simulink library "libc_hmi"  (R2015b)
settings: Solver=ode45  StartTime=0.0  StopTime=10.0  RelTol=1e-3
undefined symbols (not defined in the file or in its folder): CONST, CTRL, DiscIntNeverNeededParam
libraries: simulink x10, libc_extended_basics x4, libc_filters_diff x2
settings Model: Creator=Falkenhahn  LastModifiedBy=fav
settings DataIOCC: SaveFormat=Array  SignalLoggingSaveFormat=ModelDataLogs
settings OptimizationCC: ExpressionDepthLimit=2147483647
settings DebuggingCC: UnderspecifiedInitializationDetection=Classic  MergeDetectMultiDrivingBlocksExec=none  SolverPrmCheckMsg=warning  FcnCallInpInsideContextMsg=UseLocalSettings  StateNameClashWarn=warning
settings HardwareCC: ProdBitPerPointer=32  ProdLargestAtomicFloat=None  ProdIntDivRoundTo=Undefined  ProdEndianess=Unspecified  ProdWordSize=32  ProdHWDeviceType=32-bit Generic
settings GRTTargetCC: GeneratePreprocessorConditionals=Disable all  CombineOutputUpdateFcns=off  GRTInterface=on
settings ConfigComp: CovModelRefEnable=Off

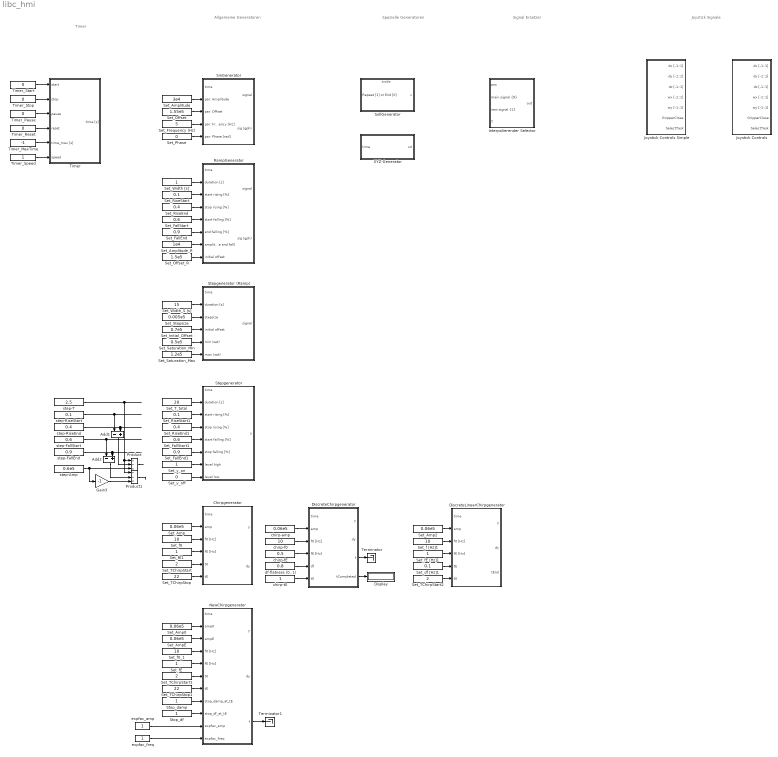
== system libc_hmi ==
  note: Timer
  note: Allgemeine
      | Generatoren
  note: Spezielle
      | Generatoren
  note: Signal
      | Ersetzer
  note: Joystick
      | Signale
  Add1 : Sum  Inputs=-+
  Add2 : Sum  Inputs=-+
  Chirpgenerator : Subsystem
      settings: AttributesFormatString=[f0,fE] >> 1/(tE-t0)
  DiscreteChirpgenerator : Subsystem
  DiscreteLinearChirpgenerator : Subsystem
  Display : Display
  Gain3 : Gain  Gain=-1
  Interpolierender Selector : Subsystem
  Joystick Controls : Subsystem  TreatAsAtomicUnit=on  SystemSampleTime=CONST.tA
      settings: AttributesFormatString=|
      | Neues Mapping mit Entprellung für BluetoothController
      | -- beachte entsprechende Einstellungen in ControlDesk --
  Joystick Controls Simple : Subsystem  TreatAsAtomicUnit=on  SystemSampleTime=CONST.tA
      settings: AttributesFormatString=|
      | Neues Mapping
      | -- beachte entsprechende --
      | -- Einstellungen in ControlDesk --
  NewChirpgenerator : Subsystem
  Product : Product  Inputs=//*
  Product1 : Product  Inputs=//*
  RampGenerator : Subsystem
  Set_Amp : Constant  Value=0.06e5
  Set_Amp0 : Constant  Value=0.06e5
  Set_Amp2 : Constant  Value=0.06e5
  Set_AmpE : Constant  Value=0.06e5
  Set_Amplitude : Constant  Value=3e4
  Set_Amplitude_R : Constant  Value=1e4
  Set_FallEnd : Constant  Value=0.9
  Set_FallEnd1 : Constant  Value=0.9
  Set_FallStart : Constant  Value=0.6
  Set_FallStart1 : Constant  Value=0.6
  Set_Frequency (Hz) : Constant  Value=5
  Set_Initial_Offset : Constant  Value=0.7e5
  Set_Offset : Constant  Value=1.55e5
  Set_Offset_R : Constant  Value=1.5e5
  Set_Phase : Constant  Value=0
  Set_RiseEnd : Constant  Value=0.4
  Set_RiseEnd1 : Constant  Value=0.4
  Set_RiseStart : Constant  Value=0.1
  Set_RiseStart1 : Constant  Value=0.1
  Set_Saturation_Max : Constant  Value=1.2e5
  Set_Saturation_Min : Constant  Value=0.5e5
  Set_Stepsize : Constant  Value=0.005e5
  Set_TChirpStart : Constant  Value=2
  Set_TChirpStart1 : Constant  Value=2
  Set_TChirpStart2 : Constant  Value=2
  Set_TChirpStop : Constant  Value=22
  Set_TChirpStop1 : Constant  Value=22
  Set_T_total : Constant  Value=20
  Set_Width [s] : Constant
  Set_Width_S [s] : Constant  Value=15
  Set_df [Hz]1 : Constant  Value=0.1
  Set_f [Hz]1 : Constant  Value=10
  Set_f0 : Constant  Value=10
  Set_f0_1 : Constant  Value=10
  "Set_fE " : Constant
  Set_fE [Hz]1 : Constant
  "Set_fE1 " : Constant
  Set_y_off : Constant  Value=0
  Set_y_on : Constant
  SinGenerator : Subsystem
  SollGenerator : Subsystem  mask(zeitgesteuerter Interpolator){len_ti=length(CTRL.LPresetTime), repext_a=1, repext_z=1}
      mask prompts: len_ti "Datenpunkte (insg)"; repext_a "Startpunkte (vorne)"; repext_z "Endpunkte (hinten)"
      mask help: Anzahl Abtastpunkte, die vorne und hinten von der Wiederholung ausgenommen sind.
      mask init:
      | last_in_loop = len_ti - repext_z;
      | first_in_loop = 1 + repext_a;
  Stepgenerator : Subsystem
  Stepgenerator (Ramp) : Subsystem  mask{pulsewidth=40}
      mask prompts: pulsewidth "Pulse width [%]"
      settings: AttributesFormatString=Puls: 0 bis %<pulsewidth> %
  Stop_damp : Constant
  Stop_df : Constant
  Terminator : Terminator
  Terminator1 : Terminator
  Timer : Subsystem
  Timer_MaxTime : Constant  Value=-1
  Timer_Pause : Constant  Value=0
  Timer_Reset : Constant  Value=0
  Timer_Speed : Constant
  Timer_Start : Constant  Value=0
  Timer_Stop : Constant  Value=0
  XYZ-Generator : Subsystem
  chirp-amp : Constant  Value=0.06e5
  chirp-f0 : Constant  Value=10
  chirp-fE : Constant  Value=0.5
  chirp-t0 : Constant
  df-flatness (0..1) : Constant  Value=0.8
  expfac_amp : Constant
      settings: AttributesFormatString=|
      | > 0.1
      | 0.5 = sqrt
      | 1 = linear
      | 2 = quadratic
  expfac_freq : Constant
      settings: AttributesFormatString=|
      | > 0.1
      | 0.5 = sqrt
      | 1 = linear
      | 2 = quadratic
  step-Amp : Constant  Value=0.6e5
  step-FallEnd : Constant  Value=0.9
  step-FallStart : Constant  Value=0.6
  step-RiseEnd : Constant  Value=0.4
  step-RiseStart : Constant  Value=0.1
  step-T : Constant  Value=2.5
  wires:
  Set_Frequency (Hz)/1 -> SinGenerator/4(par: Frequency [Hz])
  Set_Phase/1 -> SinGenerator/5(par: Phase [rad])
  Set_Offset/1 -> SinGenerator/3(par: Offset)
  Set_Amplitude/1 -> SinGenerator/2(par: Amplitude)
  Set_Width [s]/1 -> RampGenerator/2(duration [s])
  Set_FallStart/1 -> RampGenerator/5(start falling [%])
  Set_RiseEnd/1 -> RampGenerator/4(stop rising [%])
  Set_RiseStart/1 -> RampGenerator/3(start rising [%])
  Set_Amplitude_R/1 -> RampGenerator/7(amplitude (rise and fall))
  Set_FallEnd/1 -> RampGenerator/6(end falling [%])
  Set_Offset_R/1 -> RampGenerator/8(initial offset)
  Set_Saturation_Max/1 -> Stepgenerator (Ramp)/6(max (sat))
  Set_Width_S [s]/1 -> Stepgenerator (Ramp)/2(duration [s])
  Set_Initial_Offset/1 -> Stepgenerator (Ramp)/4(initial offset)
  Set_Stepsize/1 -> Stepgenerator (Ramp)/3(stepsize)
  Set_Saturation_Min/1 -> Stepgenerator (Ramp)/5(min (sat))
  Set_y_on/1 -> Stepgenerator/7(level high)
  Set_y_off/1 -> Stepgenerator/8(level low)
  Set_T_total/1 -> Stepgenerator/2(duration [s])
  Set_RiseStart1/1 -> Stepgenerator/3(start rising [%])
  Set_RiseEnd1/1 -> Stepgenerator/4(stop rising [%])
  Set_FallStart1/1 -> Stepgenerator/5(start falling [%])
  Set_FallEnd1/1 -> Stepgenerator/6(stop falling [%])
  step-RiseStart/1 -> Add1/1
  step-RiseEnd/1 -> Add1/2
  step-FallStart/1 -> Add2/1
  step-FallEnd/1 -> Add2/2
  step-T/1 -> Product/1, Product1/1
  Add1/1 -> Product/2
  Add2/1 -> Product1/2
  step-Amp/1 -> Gain3/1, Product/3
  Gain3/1 -> Product1/3
  Product/1 -> ?
  Product1/1 -> ?
  Set_Amp/1 -> Chirpgenerator/2(amp)
  Set_f0/1 -> Chirpgenerator/3(f0 [Hz])
  "Set_fE1 "/1 -> Chirpgenerator/4(fE [Hz])
  Set_TChirpStart/1 -> Chirpgenerator/5(t0)
  Set_TChirpStop/1 -> Chirpgenerator/6(tE)
  Set_Amp2/1 -> DiscreteLinearChirpgenerator/2(amp)
  Set_fE [Hz]1/1 -> DiscreteLinearChirpgenerator/4(fE [Hz])
  Set_df [Hz]1/1 -> DiscreteLinearChirpgenerator/5(tE)
  Set_f [Hz]1/1 -> DiscreteLinearChirpgenerator/3(f0 [Hz])
  Set_TChirpStart2/1 -> DiscreteLinearChirpgenerator/6(t0)
  chirp-amp/1 -> DiscreteChirpgenerator/2(amp)
  chirp-f0/1 -> DiscreteChirpgenerator/3(f0 [Hz])
  chirp-fE/1 -> DiscreteChirpgenerator/4(fE [Hz])
  df-flatness (0..1)/1 -> DiscreteChirpgenerator/5(df)
  chirp-t0/1 -> DiscreteChirpgenerator/6(t0)
  DiscreteChirpgenerator/3(f) -> Terminator/1
  DiscreteChirpgenerator/4(tCompleted) -> Display/1
  Timer_Start/1 -> Timer/1(start)
  Timer_Reset/1 -> Timer/4(reset)
  Timer_Stop/1 -> Timer/2(stop)
  Timer_MaxTime/1 -> Timer/5(time_max [s])
  Timer_Pause/1 -> Timer/3(pause)
  Timer_Speed/1 -> Timer/6(speed)
  Set_TChirpStart1/1 -> NewChirpgenerator/6(t0)
  "Set_fE "/1 -> NewChirpgenerator/5(fE [Hz])
  Set_TChirpStop1/1 -> NewChirpgenerator/7(tE)
  Set_f0_1/1 -> NewChirpgenerator/4(f0 [Hz])
  Stop_df/1 -> NewChirpgenerator/9(stop_df_at_tE)
  Stop_damp/1 -> NewChirpgenerator/8(stop_damp_at_tE)
  Set_AmpE/1 -> NewChirpgenerator/3(ampE)
  Set_Amp0/1 -> NewChirpgenerator/2(amp0)
  expfac_amp/1 -> NewChirpgenerator/10(expfac_amp)
  expfac_freq/1 -> NewChirpgenerator/11(expfac_freq)
  NewChirpgenerator/3(f) -> Terminator1/1

== system libc_hmi/Chirpgenerator ==
  time : Inport
  amp : Inport  Port=2
  f0 [Hz] : Inport  Port=3
  fE [Hz] : Inport  Port=4
  t0 : Inport  Port=5
  tE : Inport  Port=6
  Gain1 : Gain  Gain=2*pi
  Gain2 : Gain  Gain=2*pi
  steps : MATLAB Function  TreatAsAtomicUnit=on
  y : Outport
  dy : Outport  Port=2
  wires:
  steps/2(dtsin) -> dy/1
  time/1 -> steps/1(time)
  amp/1 -> steps/2(amp)
  f0 [Hz]/1 -> Gain2/1
  fE [Hz]/1 -> Gain1/1
  t0/1 -> steps/5(t0)
  tE/1 -> steps/6(tE)
  Gain1/1 -> steps/4(wE)
  Gain2/1 -> steps/3(w0)
  steps/1(rsin) -> y/1

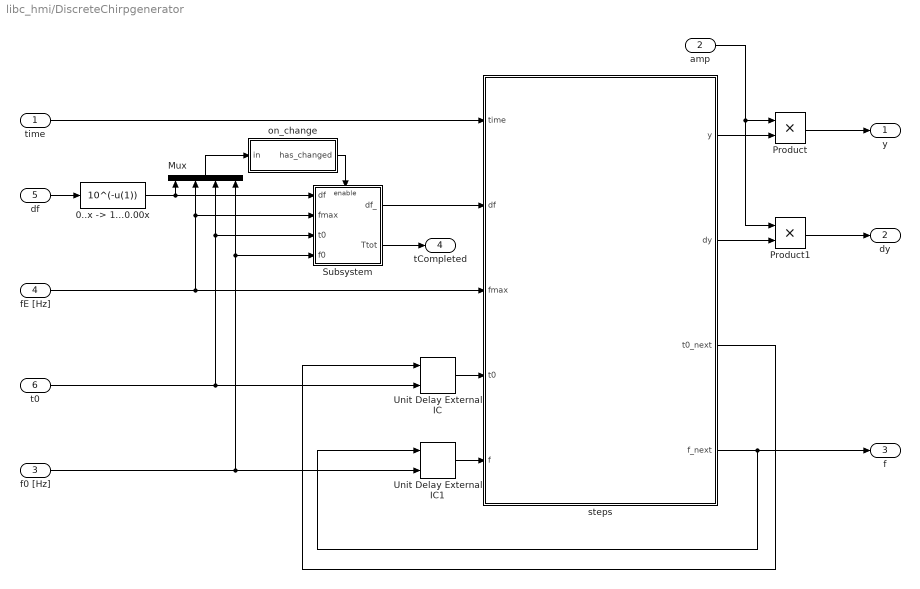
== system libc_hmi/DiscreteChirpgenerator ==
  time : Inport
  amp : Inport  Port=2
  f0 [Hz] : Inport  Port=3
  fE [Hz] : Inport  Port=4
  df : Inport  Port=5
  t0 : Inport  Port=6
  "0..x -> 1...0.00x" : Fcn  Expr=10^(-u(1))
  Mux : Mux
  Product : Product
  Product1 : Product
  Subsystem : Subsystem
  Unit Delay External IC : simulink/Additional Math & Discrete/Additional Discrete/Unit Delay External IC  tsamp=-1
  Unit Delay External IC1 : simulink/Additional Math & Discrete/Additional Discrete/Unit Delay External IC  tsamp=-1
  on_change : Subsystem
      settings: AttributesFormatString=|
      | from libl_filters_diff
      | variable frequency dependent filter
      | that has to be fixed
  steps : MATLAB Function  TreatAsAtomicUnit=on
  y : Outport
  dy : Outport  Port=2
  f : Outport  Port=3
  tCompleted : Outport  Port=4
  wires:
  "0..x -> 1...0.00x"/1 -> Mux/1, Subsystem/1(df)
  Mux/1 -> on_change/1(in)
  on_change/1(has_changed) -> Subsystem/Enable
  Subsystem/2(Ttot) -> tCompleted/1
  Subsystem/1(df_) -> steps/2(df)
  df/1 -> "0..x -> 1...0.00x"/1
  t0/1 -> Mux/3, Subsystem/3(t0), Unit Delay External IC/2
  steps/4(f_next) -> f/1, Unit Delay External IC1/1
  amp/1 -> Product1/1, Product/1
  Product1/1 -> dy/1
  steps/2(dy) -> Product1/2
  steps/1(y) -> Product/2
  fE [Hz]/1 -> Mux/2, Subsystem/2(fmax), steps/3(fmax)
  Unit Delay External IC1/1 -> steps/5(f)
  f0 [Hz]/1 -> Unit Delay External IC1/2, Mux/4, Subsystem/4(f0)
  Unit Delay External IC/1 -> steps/4(t0)
  steps/3(t0_next) -> Unit Delay External IC/1
  Product/1 -> y/1
  time/1 -> steps/1(time)

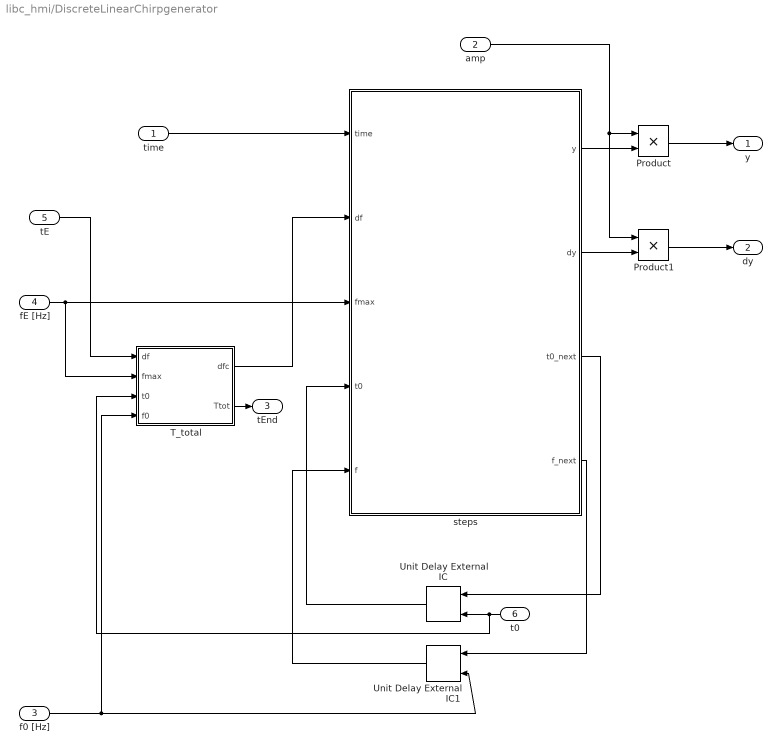
== system libc_hmi/DiscreteLinearChirpgenerator ==
  time : Inport
  amp : Inport  Port=2
  f0 [Hz] : Inport  Port=3
  fE [Hz] : Inport  Port=4
  tE : Inport  Port=5
  t0 : Inport  Port=6
  Product : Product
  Product1 : Product
  T_total : MATLAB Function  TreatAsAtomicUnit=on
  Unit Delay External IC : simulink/Additional Math & Discrete/Additional Discrete/Unit Delay External IC  tsamp=-1
  Unit Delay External IC1 : simulink/Additional Math & Discrete/Additional Discrete/Unit Delay External IC  tsamp=-1
  steps : MATLAB Function  TreatAsAtomicUnit=on
  y : Outport
  dy : Outport  Port=2
  tEnd : Outport  Port=3
  wires:
  time/1 -> steps/1(time)
  Product/1 -> y/1
  steps/3(t0_next) -> Unit Delay External IC/1
  Unit Delay External IC/1 -> steps/4(t0)
  t0/1 -> T_total/3(t0), Unit Delay External IC/2
  f0 [Hz]/1 -> T_total/4(f0), Unit Delay External IC1/2
  steps/4(f_next) -> Unit Delay External IC1/1
  Unit Delay External IC1/1 -> steps/5(f)
  tE/1 -> T_total/1(df)
  fE [Hz]/1 -> T_total/2(fmax), steps/3(fmax)
  steps/1(y) -> Product/2
  steps/2(dy) -> Product1/2
  Product1/1 -> dy/1
  amp/1 -> Product/1, Product1/1
  T_total/2(Ttot) -> tEnd/1
  T_total/1(dfc) -> steps/2(df)

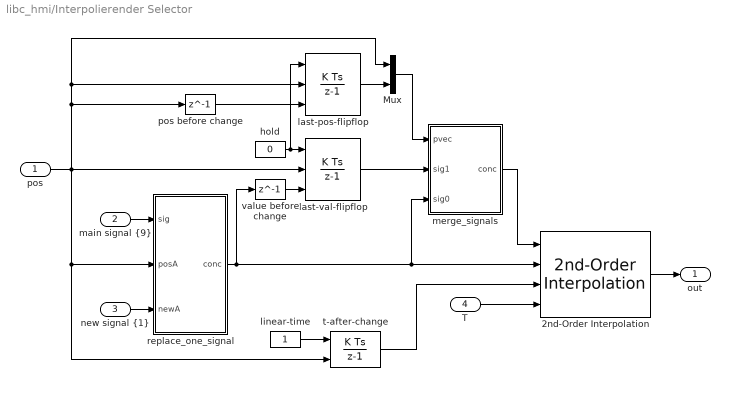
== system libc_hmi/Interpolierender Selector ==
  pos : Inport
  "main signal {9}" : Inport  Port=2
  "new signal {1}" : Inport  Port=3
  T : Inport  Port=4
  2nd-Order Interpolation : libc_filters_diff/2nd-Order Interpolation
  Mux : Mux  Inputs=2
  hold : Constant  Value=0
  last-pos-flipflop : DiscreteIntegrator  ExternalReset=either  InitialConditionSource=external  SampleTime=-1  ICPrevOutput=DiscIntNeverNeededParam  ICPrevScaledInput=DiscIntNeverNeededParam
  last-val-flipflop : DiscreteIntegrator  ExternalReset=either  InitialConditionSource=external  SampleTime=-1  ICPrevOutput=DiscIntNeverNeededParam  ICPrevScaledInput=DiscIntNeverNeededParam
  linear-time : Constant
  merge_signals : MATLAB Function  TreatAsAtomicUnit=on
  pos before change : Delay  DelayLength=1  InitialCondition=0
  replace_one_signal : MATLAB Function  TreatAsAtomicUnit=on
  t-after-change : DiscreteIntegrator  ExternalReset=either  InitialCondition=CONST.tA  SampleTime=-1  ICPrevOutput=DiscIntNeverNeededParam  ICPrevScaledInput=DiscIntNeverNeededParam
  value before change : Delay  DelayLength=1  InitialCondition=0.174
  out : Outport
  wires:
  "main signal {9}"/1 -> replace_one_signal/1(sig)
  "new signal {1}"/1 -> replace_one_signal/3(newA)
  replace_one_signal/1(conc) -> 2nd-Order Interpolation/2, merge_signals/3(sig0), value before change/1
  T/1 -> 2nd-Order Interpolation/4
  2nd-Order Interpolation/1 -> out/1
  pos/1 -> pos before change/1, last-pos-flipflop/2, Mux/1, t-after-change/2, replace_one_signal/2(posA), last-val-flipflop/2
  linear-time/1 -> t-after-change/1
  hold/1 -> last-pos-flipflop/1, last-val-flipflop/1
  value before change/1 -> last-val-flipflop/3
  last-val-flipflop/1 -> merge_signals/2(sig1)
  merge_signals/1(conc) -> 2nd-Order Interpolation/1
  t-after-change/1 -> 2nd-Order Interpolation/3
  Mux/1 -> merge_signals/1(pvec)
  last-pos-flipflop/1 -> Mux/2
  pos before change/1 -> last-pos-flipflop/3

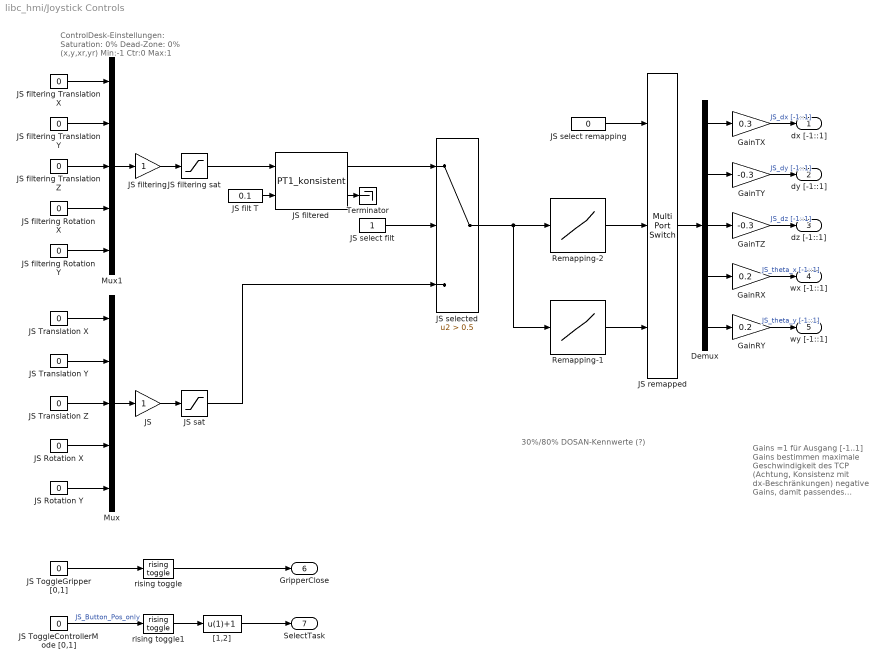
== system libc_hmi/Joystick Controls ==
  note: 30%/80% DOSAN-Kennwerte (?)
  note: Gains =1 für
      | Ausgang [-1..1]
      |
      | Gains bestimmen maximale
      | Geschwindigkeit des TCP
      | (Achtung, Konsistenz mit
      | dx-Beschränkungen)
      |
      | negative Gains,
      | damit passendes
      | Mapping für
      | stehendes
      | Welt-KoSy
  note: ControlDesk-Einstellungen:
      | Saturation: 0%
      | Dead-Zone: 0% (x,y,xr,yr)
      | Min:-1 Ctr:0 Max:1
  Demux : Demux  Outputs=5
  GainRX : Gain  Gain=0.2
  GainRY : Gain  Gain=0.2
  GainTX : Gain  Gain=0.3
  GainTY : Gain  Gain=-0.3
  GainTZ : Gain  Gain=-0.3
  JS : Gain
  JS Rotation X : Constant  Value=0  OutDataTypeStr=double
      settings: AttributesFormatString=[-1..1]
  JS Rotation Y : Constant  Value=0  OutDataTypeStr=double
      settings: AttributesFormatString=[-1..1]
  JS ToggleControllerMode [0,1] : Constant  Value=0  OutDataTypeStr=double
  JS ToggleGripper [0,1] : Constant  Value=0  OutDataTypeStr=double
  JS Translation X : Constant  Value=0  OutDataTypeStr=double
      settings: AttributesFormatString=[-1..1]
  JS Translation Y : Constant  Value=0  OutDataTypeStr=double
      settings: AttributesFormatString=[-1..1]
  JS Translation Z : Constant  Value=0  OutDataTypeStr=double
      settings: AttributesFormatString=[-1..1]
  JS filt T : Constant  Value=0.1
      settings: AttributesFormatString=|
      | 0.01: präzise, aber ruckartig
      | 0.1: weicher, dafür leicht verzögert
  JS filtered : libc_filters_diff/PT1_konsistent
  JS filtering : Gain
  JS filtering Rotation X : Constant  Value=0  OutDataTypeStr=double
      settings: AttributesFormatString=[-1..1]
  JS filtering Rotation Y : Constant  Value=0  OutDataTypeStr=double
      settings: AttributesFormatString=[-1..1]
  JS filtering Translation X : Constant  Value=0  OutDataTypeStr=double
      settings: AttributesFormatString=[-1..1]
  JS filtering Translation Y : Constant  Value=0  OutDataTypeStr=double
      settings: AttributesFormatString=[-1..1]
  JS filtering Translation Z : Constant  Value=0  OutDataTypeStr=double
      settings: AttributesFormatString=[-1..1]
  JS filtering sat : Saturate  UpperLimit=1  LowerLimit=-1
  JS remapped : MultiPortSwitch  DataPortOrder=Zero-based contiguous  Inputs=2
  JS sat : Saturate  UpperLimit=1  LowerLimit=-1
  JS select filt : Constant
      settings: AttributesFormatString=|
      | filtered input für
      | wireless controller
  JS select remapping : Constant  Value=0
  JS selected : Switch  Criteria=u2 > Threshold  Threshold=0.5
  Mux : Mux  Inputs=5
  Mux1 : Mux  Inputs=5
  Remapping-1 : Lookup_n-D  NumberOfTableDimensions=1  BreakpointsForDimension1="[-1, -0.9,  -0.301, -0.3, 0, 0.3, 0.301, 0.9, 1]"  Table=[-1, -1, -0.3, 0, 0, 0, 0.3, 1, 1]  InternalRulePriority=Speed  RndMeth=Simplest  InputSameDT=on
      settings: AttributesFormatString=|
      | Tote Zone mit
      | Losbrechsprung
      | und Plateau
  Remapping-2 : Lookup_n-D  NumberOfTableDimensions=1  BreakpointsForDimension1="[-1, -0.9,  -0.3, 0, 0.3, 0.9, 1]"  Table=[-1, -1, 0, 0, 0, 1, 1]  InternalRulePriority=Speed  RndMeth=Simplest  InputSameDT=on
      settings: AttributesFormatString=|
      | Tote Zone
      | mit Plateau
  Terminator : Terminator
  "[1,2]" : Fcn  Expr=u(1)+1
      settings: AttributesFormatString=toggle 1,2
  rising toggle : libc_extended_basics/rising toggle
  rising toggle1 : libc_extended_basics/rising toggle
  dx [-1::1] : Outport
  dy [-1::1] : Outport  Port=2
  dz [-1::1] : Outport  Port=3
  wx [-1::1] : Outport  Port=4
  wy [-1::1] : Outport  Port=5
  GripperClose : Outport  Port=6
  SelectTask : Outport  Port=7
      settings: AttributesFormatString=|
      | 0 off
      | 1 pos. only
      | 2 pos + orientation
  wires:
  JS selected/1 -> Remapping-2/1, Remapping-1/1
  JS select filt/1 -> JS selected/2
  JS sat/1 -> JS selected/3
  JS filtered/1 -> JS selected/1
  JS filtered/2 -> Terminator/1
  JS filt T/1 -> JS filtered/2
  JS filtering Translation Y/1 -> Mux1/2
  JS filtering Translation Z/1 -> Mux1/3
  JS filtering Rotation X/1 -> Mux1/4
  JS filtering Rotation Y/1 -> Mux1/5
  JS filtering sat/1 -> JS filtered/1
  JS filtering/1 -> JS filtering sat/1
  JS/1 -> JS sat/1
  Mux/1 -> JS/1
  Mux1/1 -> JS filtering/1
  JS filtering Translation X/1 -> Mux1/1
  JS Rotation Y/1 -> Mux/5
  JS Translation Y/1 -> Mux/2
  JS Translation Z/1 -> Mux/3
  JS Translation X/1 -> Mux/1
  JS Rotation X/1 -> Mux/4
  GainTX/1 -> dx [-1::1]/1  "JS_dx [-1::1]"
  GainTY/1 -> dy [-1::1]/1  "JS_dy [-1::1]"
  GainTZ/1 -> dz [-1::1]/1  "JS_dz [-1::1]"
  GainRX/1 -> wx [-1::1]/1  "JS_theta_x [-1::1]"
  GainRY/1 -> wy [-1::1]/1  "JS_theta_y [-1::1]"
  JS ToggleControllerMode [0,1]/1 -> rising toggle1/1  "JS_Button_Pos_only"
  JS ToggleGripper [0,1]/1 -> rising toggle/1
  "[1,2]"/1 -> SelectTask/1
  rising toggle/1 -> GripperClose/1
  rising toggle1/1 -> "[1,2]"/1
  Remapping-2/1 -> JS remapped/2
  Remapping-1/1 -> JS remapped/3
  JS select remapping/1 -> JS remapped/1
  JS remapped/1 -> Demux/1
  Demux/3 -> GainTZ/1
  Demux/2 -> GainTY/1
  Demux/4 -> GainRX/1
  Demux/1 -> GainTX/1
  Demux/5 -> GainRY/1

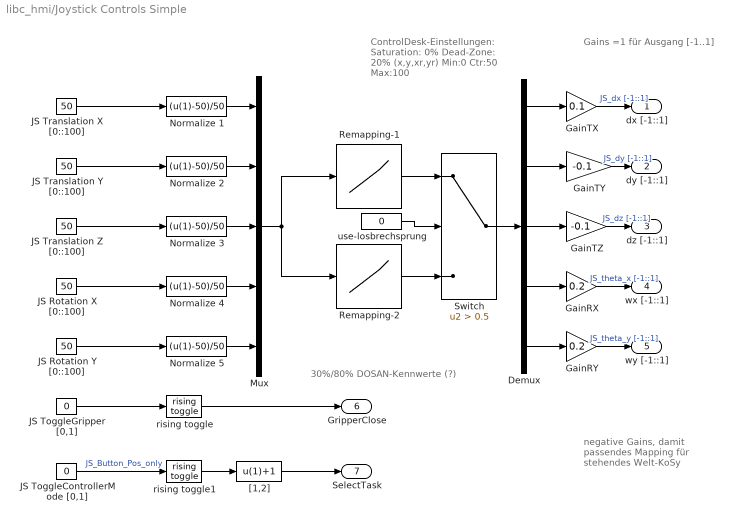
== system libc_hmi/Joystick Controls Simple ==
  note: 30%/80% DOSAN-Kennwerte (?)
  note: negative Gains,
      | damit passendes
      | Mapping für
      | stehendes
      | Welt-KoSy
  note: Gains =1 für
      | Ausgang [-1..1]
  note: ControlDesk-Einstellungen:
      | Saturation: 0%
      | Dead-Zone: 20% (x,y,xr,yr)
      | Min:0 Ctr:50 Max:100
  Demux : Demux  Outputs=5
  GainRX : Gain  Gain=0.2
  GainRY : Gain  Gain=0.2
  GainTX : Gain  Gain=0.1
  GainTY : Gain  Gain=-0.1
  GainTZ : Gain  Gain=-0.1
  JS Rotation X [0::100] : Constant  Value=50  OutDataTypeStr=double
  JS Rotation Y [0::100] : Constant  Value=50  OutDataTypeStr=double
  JS ToggleControllerMode [0,1] : Constant  Value=0  OutDataTypeStr=double
  JS ToggleGripper [0,1] : Constant  Value=0  OutDataTypeStr=double
  JS Translation X [0::100] : Constant  Value=50  OutDataTypeStr=double
  JS Translation Y [0::100] : Constant  Value=50  OutDataTypeStr=double
  JS Translation Z [0::100] : Constant  Value=50  OutDataTypeStr=double
  Mux : Mux  Inputs=5
  Normalize {1..5} (5 alike) : Fcn  Expr=(u(1)-50)/50
  Remapping-1 : Lookup_n-D  NumberOfTableDimensions=1  BreakpointsForDimension1="[-1, -0.9,  -0.301, -0.3, 0, 0.3, 0.301, 0.9, 1]"  Table=[-1, -1, -0.3, 0, 0, 0, 0.3, 1, 1]  InternalRulePriority=Speed  RndMeth=Simplest  InputSameDT=on
      settings: AttributesFormatString=|
      | Tote Zone mit
      | Losbrechsprung
      | und Plateau
  Remapping-2 : Lookup_n-D  NumberOfTableDimensions=1  BreakpointsForDimension1="[-1, -0.9,  -0.3, 0, 0.3, 0.9, 1]"  Table=[-1, -1, 0, 0, 0, 1, 1]  InternalRulePriority=Speed  RndMeth=Simplest  InputSameDT=on
      settings: AttributesFormatString=|
      | Tote Zone
      | mit Plateau
  Switch : Switch  Criteria=u2 > Threshold  Threshold=0.5
  "[1,2]" : Fcn  Expr=u(1)+1
      settings: AttributesFormatString=toggle 1,2
  rising toggle : libc_extended_basics/rising toggle
  rising toggle1 : libc_extended_basics/rising toggle
  use-losbrechsprung : Constant  Value=0
  dx [-1::1] : Outport
  dy [-1::1] : Outport  Port=2
  dz [-1::1] : Outport  Port=3
  wx [-1::1] : Outport  Port=4
  wy [-1::1] : Outport  Port=5
  GripperClose : Outport  Port=6
  SelectTask : Outport  Port=7
      settings: AttributesFormatString=|
      | 0 off
      | 1 pos. only
      | 2 pos + orientation
  wires:
  JS Translation X [0::100]/1 -> Normalize 1/1
  JS Translation Y [0::100]/1 -> Normalize 2/1
  JS Translation Z [0::100]/1 -> Normalize 3/1
  JS Rotation X [0::100]/1 -> Normalize 4/1
  JS Rotation Y [0::100]/1 -> Normalize 5/1
  GainTX/1 -> dx [-1::1]/1  "JS_dx [-1::1]"
  GainTY/1 -> dy [-1::1]/1  "JS_dy [-1::1]"
  GainTZ/1 -> dz [-1::1]/1  "JS_dz [-1::1]"
  GainRX/1 -> wx [-1::1]/1  "JS_theta_x [-1::1]"
  GainRY/1 -> wy [-1::1]/1  "JS_theta_y [-1::1]"
  JS ToggleControllerMode [0,1]/1 -> rising toggle1/1  "JS_Button_Pos_only"
  JS ToggleGripper [0,1]/1 -> rising toggle/1
  "[1,2]"/1 -> SelectTask/1
  rising toggle/1 -> GripperClose/1
  rising toggle1/1 -> "[1,2]"/1
  Normalize 3/1 -> Mux/3
  Normalize 2/1 -> Mux/2
  Normalize 4/1 -> Mux/4
  Normalize 1/1 -> Mux/1
  Normalize 5/1 -> Mux/5
  Mux/1 -> Remapping-1/1, Remapping-2/1
  Remapping-2/1 -> Switch/3
  Remapping-1/1 -> Switch/1
  use-losbrechsprung/1 -> Switch/2
  Switch/1 -> Demux/1
  Demux/3 -> GainTZ/1
  Demux/2 -> GainTY/1
  Demux/4 -> GainRX/1
  Demux/1 -> GainTX/1
  Demux/5 -> GainRY/1

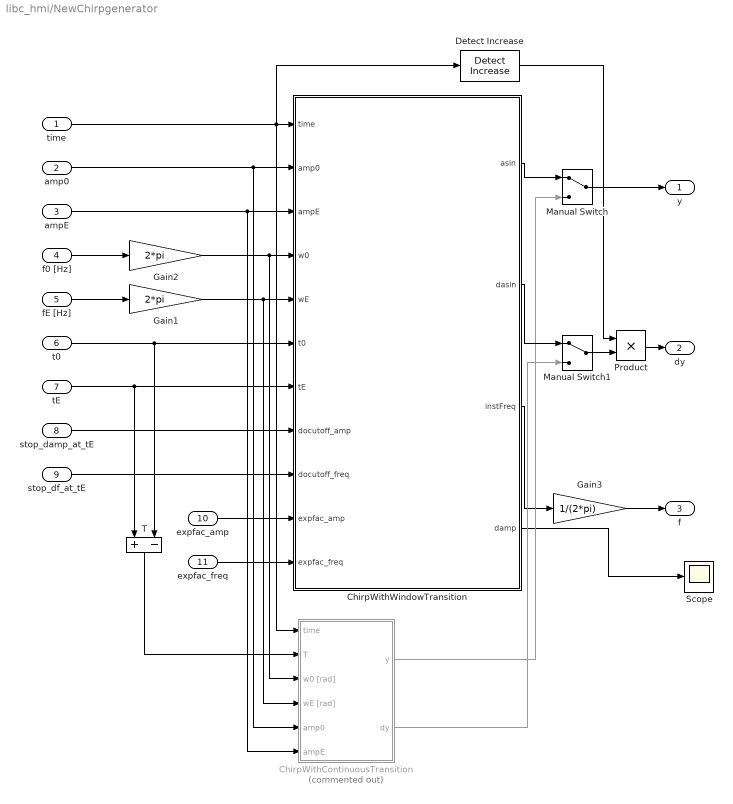
== system libc_hmi/NewChirpgenerator ==
  time : Inport
  amp0 : Inport  Port=2
  ampE : Inport  Port=3
  f0 [Hz] : Inport  Port=4
  fE [Hz] : Inport  Port=5
  t0 : Inport  Port=6
  tE : Inport  Port=7
  stop_damp_at_tE : Inport  Port=8
  stop_df_at_tE : Inport  Port=9
  expfac_amp : Inport  Port=10
  expfac_freq : Inport  Port=11
  ChirpWithContinuousTransition : Subsystem  Commented=on
  ChirpWithWindowTransition : MATLAB Function  TreatAsAtomicUnit=on
      settings: AttributesFormatString=allows: amp0=ampE & w0=wE
  Detect Increase : simulink/Logic and Bit Operations/Detect Increase  vinit=-1.0  InputProcessing=Inherited  OutDataTypeStr=boolean
  Gain1 : Gain  Gain=2*pi
  Gain2 : Gain  Gain=2*pi
  Gain3 : Gain  Gain=1/(2*pi)
  Manual Switch : ManualSwitch
  Manual Switch1 : ManualSwitch
  Product : Product
  Scope : Scope
  T : Sum  Inputs=+-
  y : Outport
  dy : Outport  Port=2
  f : Outport  Port=3
  wires:
  ChirpWithWindowTransition/4(damp) -> Scope/1
  expfac_amp/1 -> ChirpWithWindowTransition/10(expfac_amp)
  Detect Increase/1 -> Product/1
  Product/1 -> dy/1
  Gain3/1 -> f/1
  ChirpWithWindowTransition/3(instFreq) -> Gain3/1
  expfac_freq/1 -> ChirpWithWindowTransition/11(expfac_freq)
  stop_df_at_tE/1 -> ChirpWithWindowTransition/9(docutoff_freq)
  stop_damp_at_tE/1 -> ChirpWithWindowTransition/8(docutoff_amp)
  Gain2/1 -> ChirpWithWindowTransition/4(w0), ChirpWithContinuousTransition/3(w0 [rad])
  Gain1/1 -> ChirpWithWindowTransition/5(wE), ChirpWithContinuousTransition/4(wE [rad])
  tE/1 -> ChirpWithWindowTransition/7(tE), T/1
  t0/1 -> ChirpWithWindowTransition/6(t0), T/2
  fE [Hz]/1 -> Gain1/1
  f0 [Hz]/1 -> Gain2/1
  amp0/1 -> ChirpWithWindowTransition/2(amp0), ChirpWithContinuousTransition/5(amp0)
  time/1 -> ChirpWithContinuousTransition/1(time), ChirpWithWindowTransition/1(time), Detect Increase/1
  ampE/1 -> ChirpWithWindowTransition/3(ampE), ChirpWithContinuousTransition/6(ampE)
  T/1 -> ChirpWithContinuousTransition/2(T)
  ChirpWithWindowTransition/1(asin) -> Manual Switch/1
  Manual Switch/1 -> y/1
  ChirpWithContinuousTransition/1(y) -> Manual Switch/2
  ChirpWithWindowTransition/2(dasin) -> Manual Switch1/1
  Manual Switch1/1 -> Product/2
  ChirpWithContinuousTransition/2(dy) -> Manual Switch1/2

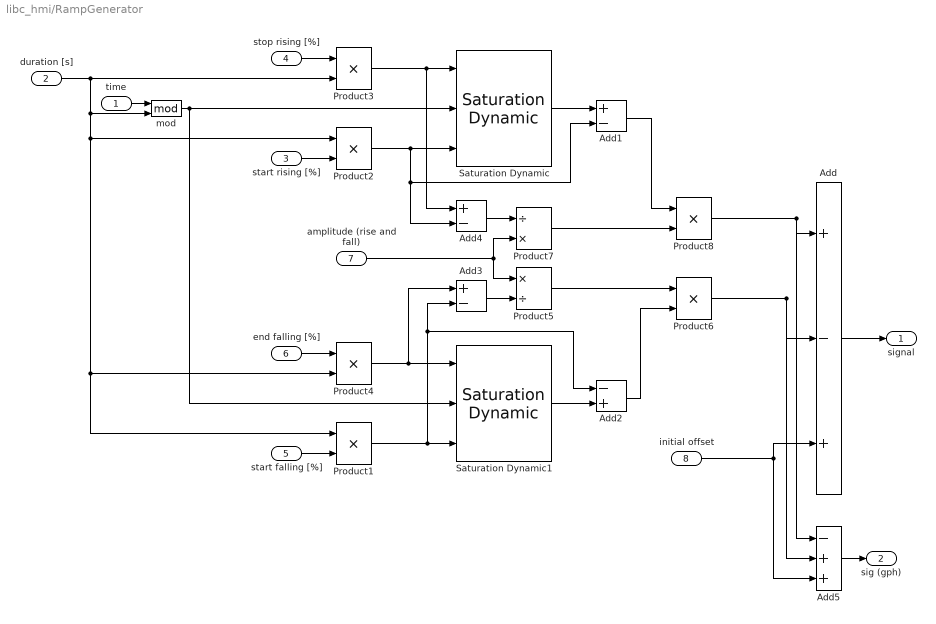
== system libc_hmi/RampGenerator ==
  time : Inport
  duration [s] : Inport  Port=2
  start rising [%] : Inport  Port=3
  stop rising [%] : Inport  Port=4
  start falling [%] : Inport  Port=5
  end falling [%] : Inport  Port=6
  amplitude (rise and fall) : Inport  Port=7
  initial offset : Inport  Port=8
  Add : Sum  Inputs=+-|+
  Add1 : Sum  Inputs=+-
  Add2 : Sum  Inputs=-+
  Add3 : Sum  Inputs=+-
  Add4 : Sum  Inputs=+-
  Add5 : Sum  Inputs=-++
  Product{1..4,6,8} (6 alike) : Product  RndMeth=Zero
  Product5 : Product  Inputs=*/  RndMeth=Zero
  Product7 : Product  Inputs=/*  RndMeth=Zero
  Saturation Dynamic : simulink/Discontinuities/Saturation Dynamic  OutMin=[]  OutMax=[]  OutDataTypeStr=Inherit: Same as second input  OutDataType=fixdt(1, 16)  OutScaling=2^-10  DoSatur=off
  Saturation Dynamic1 : simulink/Discontinuities/Saturation Dynamic  OutMin=[]  OutMax=[]  OutDataTypeStr=Inherit: Same as second input  OutDataType=fixdt(1, 16)  OutScaling=2^-10  DoSatur=off
  mod : Math  Operator=mod  SaturateOnIntegerOverflow=on
  signal : Outport
  sig (gph) : Outport  Port=2
  wires:
  duration [s]/1 -> Product3/2, Product2/1, Product4/2, Product1/1, mod/2
  Product2/1 -> Add1/2, Add4/2, Saturation Dynamic/3
  Product3/1 -> Add4/1, Saturation Dynamic/1
  start rising [%]/1 -> Product2/2
  stop rising [%]/1 -> Product3/1
  mod/1 -> Saturation Dynamic1/2, Saturation Dynamic/2
  Product1/1 -> Add3/2, Add2/1, Saturation Dynamic1/3
  Product4/1 -> Add3/1, Saturation Dynamic1/1
  start falling [%]/1 -> Product1/2
  end falling [%]/1 -> Product4/1
  Saturation Dynamic/1 -> Add1/1
  Saturation Dynamic1/1 -> Add2/2
  Product8/1 -> Add5/1, Add/1
  Product6/1 -> Add5/2, Add/2
  Add3/1 -> Product5/2
  amplitude (rise and fall)/1 -> Product5/1, Product7/2
  Product5/1 -> Product6/1
  Add2/1 -> Product6/2
  Add4/1 -> Product7/1
  Add1/1 -> Product8/1
  Product7/1 -> Product8/2
  initial offset/1 -> Add5/3, Add/3
  Add/1 -> signal/1
  time/1 -> mod/1
  Add5/1 -> sig (gph)/1

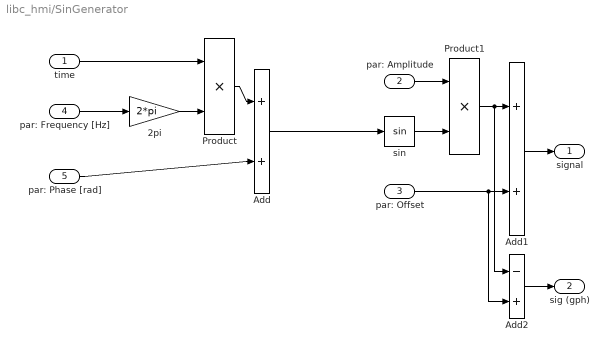
== system libc_hmi/SinGenerator ==
  time : Inport
  par: Amplitude : Inport  Port=2
  par: Offset : Inport  Port=3
  par: Frequency [Hz] : Inport  Port=4
  par: Phase [rad] : Inport  Port=5
  2pi : Gain  Gain=2*pi
  Add : Sum  Inputs=+||+
  Add1 : Sum
  Add2 : Sum  Inputs=-+
  Product : Product  RndMeth=Zero
  Product1 : Product  RndMeth=Zero
  sin : Trigonometry
  signal : Outport
  sig (gph) : Outport  Port=2
  wires:
  par: Frequency [Hz]/1 -> 2pi/1
  2pi/1 -> Product/2
  time/1 -> Product/1
  Product/1 -> Add/1
  par: Phase [rad]/1 -> Add/2
  Add/1 -> sin/1
  sin/1 -> Product1/2
  Product1/1 -> Add2/1, Add1/1
  par: Amplitude/1 -> Product1/1
  par: Offset/1 -> Add2/2, Add1/2
  Add1/1 -> signal/1
  Add2/1 -> sig (gph)/1

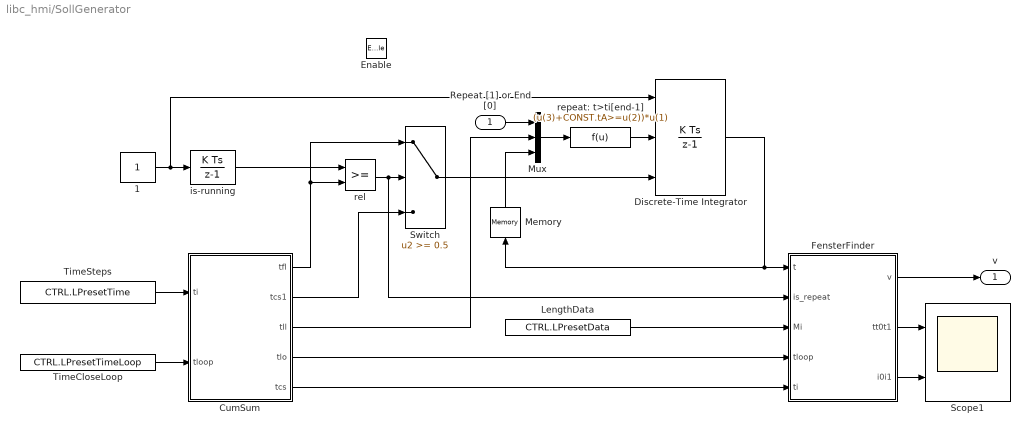
== system libc_hmi/SollGenerator ==
  Repeat [1] or End [0] : Inport
  Enable : EnablePort  StatesWhenEnabling=reset
  1 : Constant
  CumSum : MATLAB Function  TreatAsAtomicUnit=on
  Discrete-Time Integrator : DiscreteIntegrator  gainval=1  ExternalReset=rising  InitialConditionSource=external  SampleTime=CONST.tA  ICPrevOutput=DiscIntNeverNeededParam  ICPrevScaledInput=DiscIntNeverNeededParam
  FensterFinder : MATLAB Function  TreatAsAtomicUnit=on
  LengthData : Constant  Value=CTRL.LPresetData  OutDataTypeStr=Inherit: Inherit via back propagation  SampleTime=CONST.tA
  Memory : Memory  InheritSampleTime=on
  Mux : Mux  Inputs=3
  Scope1 : Scope  NumInputPorts=2
  Switch : Switch  Threshold=0.5
  TimeCloseLoop : Constant  Value=CTRL.LPresetTimeLoop  OutDataTypeStr=Inherit: Inherit via back propagation  SampleTime=CONST.tA
  TimeSteps : Constant  Value=CTRL.LPresetTime  OutDataTypeStr=Inherit: Inherit via back propagation  SampleTime=CONST.tA
  is-running : DiscreteIntegrator  gainval=1  SampleTime=CONST.tA  ICPrevOutput=DiscIntNeverNeededParam  ICPrevScaledInput=DiscIntNeverNeededParam
  rel : RelationalOperator  OutDataTypeStr=boolean
  repeat: t>ti[end-1] : Fcn  Expr=(u(3)+CONST.tA>=u(2))*u(1)
  v : Outport
  wires:
  FensterFinder/2(tt0t1) -> Scope1/1
  FensterFinder/3(i0i1) -> Scope1/2
  Memory/1 -> Mux/3
  CumSum/3(tll) -> Mux/2
  CumSum/4(tlo) -> FensterFinder/4(tloop)
  TimeCloseLoop/1 -> CumSum/2(tloop)
  TimeSteps/1 -> CumSum/1(ti)
  CumSum/5(tcs) -> FensterFinder/5(ti)
  rel/1 -> Switch/2, FensterFinder/2(is_repeat)
  Repeat [1] or End [0]/1 -> Mux/1
  FensterFinder/1(v) -> v/1
  LengthData/1 -> FensterFinder/3(Mi)
  repeat: t>ti[end-1]/1 -> Discrete-Time Integrator/2
  is-running/1 -> rel/1
  CumSum/1(tfl) -> rel/2, Switch/1
  CumSum/2(tcs1) -> Switch/3
  Mux/1 -> repeat: t>ti[end-1]/1
  Discrete-Time Integrator/1 -> Memory/1, FensterFinder/1(t)
  1/1 -> is-running/1, Discrete-Time Integrator/1
  Switch/1 -> Discrete-Time Integrator/3

== system libc_hmi/Stepgenerator ==
  time : Inport
  duration [s] : Inport  Port=2
  start rising [%] : Inport  Port=3
  stop rising [%] : Inport  Port=4
  start falling [%] : Inport  Port=5
  stop falling [%] : Inport  Port=6
  level high : Inport  Port=7
  level low : Inport  Port=8
  Product{,1..3} (4 alike) : Product
  steps : MATLAB Function  TreatAsAtomicUnit=on
  y : Outport
  wires:
  time/1 -> steps/1(time)
  duration [s]/1 -> Product3/2, Product2/2, Product1/2, Product/2, steps/8(Tmax)
  steps/1(y) -> y/1
  start rising [%]/1 -> Product/1
  Product/1 -> steps/4(T_high_start)
  stop falling [%]/1 -> Product3/1
  start falling [%]/1 -> Product2/1
  stop rising [%]/1 -> Product1/1
  Product1/1 -> steps/5(T_high_stop)
  Product2/1 -> steps/6(T_low_start)
  Product3/1 -> steps/7(T_low_stop)
  level high/1 -> steps/2(yon)
  level low/1 -> steps/3(yoff)

== system libc_hmi/Stepgenerator (Ramp) ==
  time : Inport
  duration [s] : Inport  Port=2
  stepsize : Inport  Port=3
  initial offset : Inport  Port=4
  min (sat) : Inport  Port=5
  max (sat) : Inport  Port=6
  Add : Sum  Inputs=+|+
  Fcn : Fcn  Expr=floor(u(1))
  Product : Product  RndMeth=Zero
  Product1 : Product  Inputs=*/  RndMeth=Zero
  Product2 : Product  Inputs=**  RndMeth=Zero
  Pulse Generator : DiscretePulseGenerator  PulseType=Time based  TimeSource=Use external signal  Period=1  PulseWidth=pulsewidth
  Saturation Dynamic : simulink/Discontinuities/Saturation Dynamic  OutMin=[]  OutMax=[]  OutDataTypeStr=Inherit: Same as second input  OutDataType=fixdt(1, 16)  OutScaling=2^-10  DoSatur=off
  signal : Outport
  wires:
  Saturation Dynamic/1 -> signal/1
  max (sat)/1 -> Saturation Dynamic/1
  min (sat)/1 -> Saturation Dynamic/3
  initial offset/1 -> Add/2
  stepsize/1 -> Product2/2
  duration [s]/1 -> Product1/2
  Product1/1 -> Fcn/1, Pulse Generator/1
  Pulse Generator/1 -> Product/1
  Fcn/1 -> Product/2
  Add/1 -> Saturation Dynamic/2
  time/1 -> Product1/1
  Product/1 -> Product2/1
  Product2/1 -> Add/1

== system libc_hmi/Timer ==
  start : Inport
  stop : Inport  Port=2
  pause : Inport  Port=3
  reset : Inport  Port=4
  time_max [s] : Inport  Port=5
  speed : Inport  Port=6
  0 speed if pause : Fcn  Expr=(u(1)<0.5)*u(2)
  Logik : Subsystem
  Mux : Mux  Inputs=2
  timer : Subsystem
  time [s] : Outport
  wires:
  pause/1 -> Mux/1
  speed/1 -> Mux/2
  Mux/1 -> 0 speed if pause/1
  0 speed if pause/1 -> timer/1(speed_factor)
  time_max [s]/1 -> Logik/4(time_max)
  reset/1 -> Logik/3(reset)
  stop/1 -> Logik/2(stop)
  start/1 -> Logik/1(start)
  Logik/2(time_reset) -> timer/2(time_reset)
  Logik/1(enable) -> timer/Enable
  timer/1(time) -> time [s]/1, Logik/5(time)  "time"

== system libc_hmi/XYZ-Generator ==
  time : Inport
  Dreieck : MATLAB Function  TreatAsAtomicUnit=on
  Mux : Mux  Inputs=3
  t1 : Constant  Value=3.5  OutDataTypeStr=Inherit: Inherit via back propagation  SampleTime=CONST.tA
  t2 : Constant  Value=8  OutDataTypeStr=Inherit: Inherit via back propagation  SampleTime=CONST.tA
  x0 : Constant  Value=-0.1  OutDataTypeStr=Inherit: Inherit via back propagation  SampleTime=CONST.tA
  x1 : Constant  Value=0.1  OutDataTypeStr=Inherit: Inherit via back propagation  SampleTime=CONST.tA
  y : Constant  Value=0  OutDataTypeStr=Inherit: Inherit via back propagation  SampleTime=CONST.tA
  z0 : Constant  Value=0.6  OutDataTypeStr=Inherit: Inherit via back propagation  SampleTime=CONST.tA
  z2 : Constant  Value=0.75  OutDataTypeStr=Inherit: Inherit via back propagation  SampleTime=CONST.tA
  xd : Outport
  wires:
  t2/1 -> Dreieck/2(t2)
  t1/1 -> Dreieck/6(t1)
  time/1 -> Dreieck/1(t)
  Dreieck/1(x) -> Mux/1
  y/1 -> Mux/2
  Dreieck/2(z) -> Mux/3
  x0/1 -> Dreieck/3(x0)
  z2/1 -> Dreieck/7(z2)
  z0/1 -> Dreieck/4(z0)
  x1/1 -> Dreieck/5(x1)
  Mux/1 -> xd/1

== system libc_hmi/DiscreteChirpgenerator/Subsystem ==
  df : Inport
  fmax : Inport  Port=2
  t0 : Inport  Port=3
  f0 : Inport  Port=4
  Enable : EnablePort
  T_total : MATLAB Function  TreatAsAtomicUnit=on
  df_ : Outport
  Ttot : Outport  Port=2
  wires:
  t0/1 -> T_total/3(t0)
  f0/1 -> T_total/4(f0)
  fmax/1 -> T_total/2(fmax)
  T_total/1(df_) -> df_/1
  T_total/2(Ttot) -> Ttot/1
  df/1 -> T_total/1(df)

== system libc_hmi/DiscreteChirpgenerator/on_change ==
  in : Inport
  not equal : RelationalOperator  Operator=~=  OutDataTypeStr=boolean
  old : UnitDelay  InitialCondition=-1  SampleTime=-1
  has_changed : Outport
  wires:
  not equal/1 -> has_changed/1
  old/1 -> not equal/2
  in/1 -> old/1, not equal/1

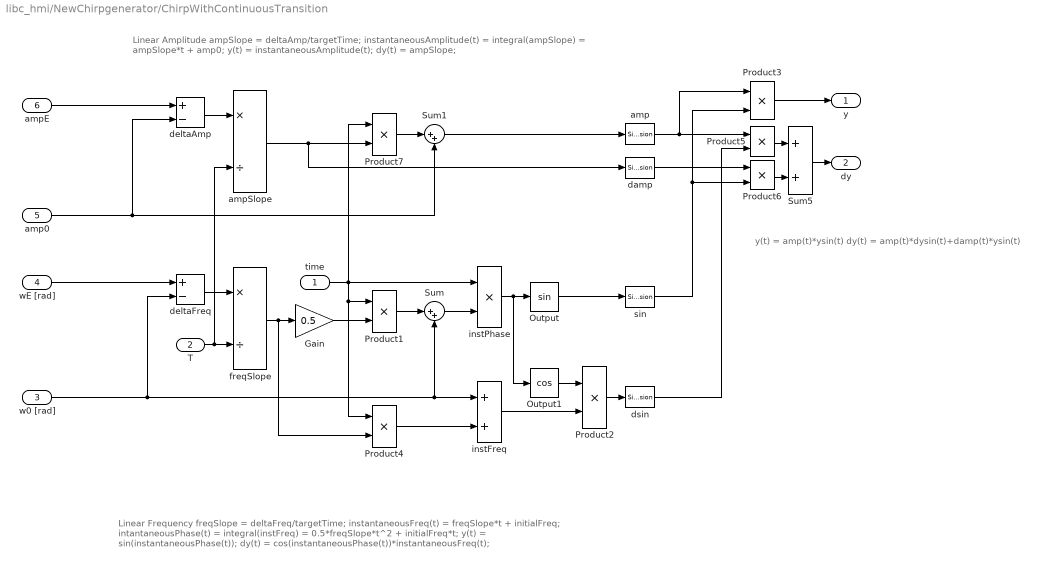
== system libc_hmi/NewChirpgenerator/ChirpWithContinuousTransition ==
  note: Linear Amplitude
      |
      | ampSlope = deltaAmp/targetTime;
      | instantaneousAmplitude(t) = integral(ampSlope) = ampSlope*t + amp0;
      | y(t)  = instantaneousAmplitude(t);
      | dy(t) = ampSlope;
  note: y(t)  = amp(t)*ysin(t)
      | dy(t) = amp(t)*dysin(t)+damp(t)*ysin(t)
  note: Linear Frequency
      |
      | freqSlope = deltaFreq/targetTime;
      | instantaneousFreq(t) = freqSlope*t + initialFreq;
      | intantaneousPhase(t) = integral(instFreq) = 0.5*freqSlope*t^2 + initialFreq*t;
      | y(t)  = sin(instantaneousPhase(t));
      | dy(t) = cos(instantaneousPhase(t))*instantaneousFreq(t);
  time : Inport
  T : Inport  Port=2
      settings: AttributesFormatString=targetTime
  w0 [rad] : Inport  Port=3
      settings: AttributesFormatString=initialFrequency
  wE [rad] : Inport  Port=4
      settings: AttributesFormatString=finalFrequency
  amp0 : Inport  Port=5
  ampE : Inport  Port=6
  Gain : Gain  DisableCoverage=on  Gain=0.5  OutDataTypeStr=Inherit: Same as input  ParamDataTypeStr=Inherit: Same as input
  Output : Trigonometry
      settings: AttributesFormatString=sin
  Output1 : Trigonometry  Operator=cos
  Product{1..7} (7 alike) : Product  DisableCoverage=on  SaturateOnIntegerOverflow=on  InputSameDT=on  OutDataTypeStr=Inherit: Same as first input
      Product2 settings: AttributesFormatString=dsin
  Sum : Sum  DisableCoverage=on  Inputs=|++  SaturateOnIntegerOverflow=on  InputSameDT=on  OutDataTypeStr=Inherit: Same as first input
  Sum1 : Sum  DisableCoverage=on  Inputs=|++  SaturateOnIntegerOverflow=on  InputSameDT=on  OutDataTypeStr=Inherit: Same as first input
  Sum5 : Sum
  amp : SignalConversion
  ampSlope : Product  DisableCoverage=on  Inputs=*/  SaturateOnIntegerOverflow=on  InputSameDT=on  OutDataTypeStr=Inherit: Same as first input
  damp : SignalConversion
  deltaAmp : Sum  Inputs=+-
  deltaFreq : Sum  Inputs=+-
  dsin : SignalConversion
  freqSlope : Product  DisableCoverage=on  Inputs=*/  SaturateOnIntegerOverflow=on  InputSameDT=on  OutDataTypeStr=Inherit: Same as first input
  instFreq : Sum
  instPhase : Product  DisableCoverage=on  SaturateOnIntegerOverflow=on  InputSameDT=on  OutDataTypeStr=Inherit: Same as first input
  sin : SignalConversion
  y : Outport
  dy : Outport  Port=2
  wires:
  Product2/1 -> dsin/1
  sin/1 -> Product3/2, Product6/2
  damp/1 -> Product6/1
  amp/1 -> Product5/1, Product3/1
  Product7/1 -> Sum1/1
  amp0/1 -> deltaAmp/2, Sum1/2
  ampE/1 -> deltaAmp/1
  deltaAmp/1 -> ampSlope/1
  ampSlope/1 -> Product7/2, damp/1
  Sum1/1 -> amp/1
  Sum5/1 -> dy/1
  Product6/1 -> Sum5/2
  Product5/1 -> Sum5/1
  Product3/1 -> y/1
  Product4/1 -> instFreq/2
  instFreq/1 -> Product2/2
  Output1/1 -> Product2/1
  dsin/1 -> Product5/2
  Output/1 -> sin/1
  wE [rad]/1 -> deltaFreq/1
  deltaFreq/1 -> freqSlope/1
  w0 [rad]/1 -> Sum/2, instFreq/1, deltaFreq/2
  T/1 -> freqSlope/2, ampSlope/2
  Sum/1 -> instPhase/2
  instPhase/1 -> Output/1, Output1/1
  Gain/1 -> Product1/2
  freqSlope/1 -> Gain/1, Product4/2
  time/1 -> instPhase/1, Product7/1, Product1/1, Product4/1
  Product1/1 -> Sum/1

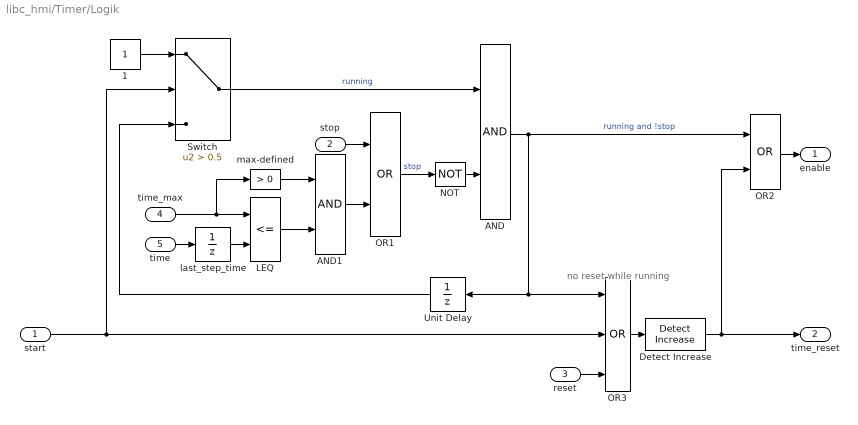
== system libc_hmi/Timer/Logik ==
  note: no reset
      | while running
  start : Inport
  stop : Inport  Port=2
  reset : Inport  Port=3
  time_max : Inport  Port=4
  time : Inport  Port=5
  1 : Constant
  AND : Logic  AllPortsSameDT=off  OutDataTypeStr=boolean
  AND1 : Logic  AllPortsSameDT=off  OutDataTypeStr=boolean
  Detect Increase : simulink/Logic and Bit Operations/Detect Increase  vinit=0.0  InputProcessing=Inherited  OutDataTypeStr=uint8
  LEQ : RelationalOperator  Operator=<=  OutDataTypeStr=boolean
  NOT : Logic  Operator=NOT  AllPortsSameDT=off  OutDataTypeStr=boolean
  OR1 : Logic  Operator=OR  AllPortsSameDT=off  OutDataTypeStr=boolean
  OR2 : Logic  Operator=OR  AllPortsSameDT=off  OutDataTypeStr=boolean
  OR3 : Logic  Operator=OR  Inputs=3  AllPortsSameDT=off  OutDataTypeStr=boolean
  Switch : Switch  Criteria=u2 > Threshold  Threshold=0.5
  Unit Delay : UnitDelay  SampleTime=-1
  last_step_time : UnitDelay  SampleTime=-1
  max-defined : simulink/Logic and Bit Operations/Compare To Constant  relop=>  const=0  OutDataTypeStr=boolean
  enable : Outport
  time_reset : Outport  Port=2
  wires:
  max-defined/1 -> AND1/1
  LEQ/1 -> AND1/2
  AND1/1 -> OR1/2
  reset/1 -> OR3/3
  Detect Increase/1 -> OR2/2, time_reset/1
  OR3/1 -> Detect Increase/1
  start/1 -> OR3/2, Switch/2
  OR2/1 -> enable/1
  AND/1 -> OR2/1, Unit Delay/1, OR3/1  "running and !stop"
  time/1 -> last_step_time/1
  time_max/1 -> LEQ/1, max-defined/1
  stop/1 -> OR1/1
  last_step_time/1 -> LEQ/2
  Switch/1 -> AND/1  "running"
  NOT/1 -> AND/2
  Unit Delay/1 -> Switch/3
  1/1 -> Switch/1
  OR1/1 -> NOT/1  "stop"

== system libc_hmi/Timer/timer ==
  speed_factor : Inport
  time_reset : Inport  Port=2
  Enable : EnablePort  StatesWhenEnabling=reset
  Discrete-Time Integrator : DiscreteIntegrator  ExternalReset=level  SampleTime=-1  ICPrevOutput=DiscIntNeverNeededParam  ICPrevScaledInput=DiscIntNeverNeededParam
  time : Outport  InitialOutput=0
  wires:
  time_reset/1 -> Discrete-Time Integrator/2
  Discrete-Time Integrator/1 -> time/1
  speed_factor/1 -> Discrete-Time Integrator/1

== matlab function libc_hmi/SollGenerator/CumSum ==
  data: tfl output; tcs1 output; tll output; tlo output; tcs output; ti input; first_in_loop parameter; last_in_loop parameter; tloop input
function [tfl,tcs1,tll,tlo,tcs] = mod(ti, first_in_loop, last_in_loop, tloop)
%#codegen

    tlo = tloop;
    tcs = cumsum(ti);
    tcs1 = tcs(1);
    tll = tcs(last_in_loop)+tlo;
    tfl = tcs(first_in_loop); 

   
end

== matlab function libc_hmi/Interpolierender Selector/merge_signals ==
  data: pvec input; sig1 input; sig0 input; conc output
function conc = replsig(pvec, sig1, sig0)

    n = 9;
    
    pvec = round(pvec); % Sicherheitsmaßnahme
    
    selector = zeros(9,1);
    for i=1:length(pvec)
        if pvec(i) > 0 && pvec(i) <= n
            selector(pvec(i)) = 1;
        end
    end

    conc = sig0;
    for i=1:n
       if selector(i) == 1
           conc(i) = sig1(i);
       end
    end
end

== matlab function libc_hmi/SollGenerator/FensterFinder ==
  data: t input; is_repeat input; Mi input; tloop input; v output size=9; ti input; repext_a parameter; last_in_loop parameter; tt0t1 output; i0i1 output
function [v, tt0t1, i0i1] = C1(t, is_repeat, Mi, tloop, ti, repext_a, last_in_loop)
%#codegen

    %% Parameter

    teps = 1e-6;

    %% Begrenzung

    if t <= ti(1)
        t = ti(1)+teps;
    elseif t > ti(end)
        t = ti(end);
    end

    %% Fensterauswahl

    tmp = find(ti-t>0, 1 );
    if length(tmp) < 1
        i1 = length(ti);
    else
        i1 = tmp(1,1);
        if i1 <= 1
            i1 = 2;
        elseif i1 > last_in_loop && is_repeat
            i1 = repext_a + 1;
        end
    end

    i0 = i1-1;
    if i0 <= repext_a && is_repeat
        i0 = last_in_loop;

        t0 = ti(i0);
        t1 = t0+tloop;
    else
        t0 = ti(i0);
        t1 = ti(i1);
    end
    
    %% Datensatz abgreifen
    
    x0vec = Mi(:,i0);
    x1vec = Mi(:,i1);    
    
    %% Algorithmus

    if abs(t-t0) < teps
        v = x0vec; 
    elseif abs(t-t1) < teps
        v = x1vec;
    else
    
        %% C1-Interpolation mit Polynom dritter Ordnung.
        d = x0vec;
        c = 0;
        a = -2*(x1vec-x0vec)/(t1-t0)^3;
        b =  3*(x1vec-x0vec)/(t1-t0)^2;

        v = a*(t-t0).^3 + b*(t-t0).^2 + c*(t-t0) + d;

    end;
    
    
    tt0t1 = [t0 t t1];
    i0i1 = [i0 i1];
    % x = [x0vec(1), v(1), x1vec(1)];
    
end

== matlab function libc_hmi/Interpolierender Selector/replace_one_signal ==
  data: sig input; conc output; posA input; newA input
function conc = replsig(sig, posA, newA)

    posA = floor(posA);

    conc = sig;
    if posA > 0
        if posA > length(sig)
            posA = length(sig);
        end
        conc(posA) = newA;
    end

end

== matlab function libc_hmi/Stepgenerator/steps ==
  data: time input; y output; yon input; yoff input; T_high_start input; T_high_stop input; T_low_start input; T_low_stop input; Tmax input
function y = step(time, yon, yoff, T_high_start, T_high_stop, T_low_start, T_low_stop, Tmax)
%#codegen

t = mod(time,Tmax);

y = 0;
if t >= T_high_start && t < T_high_stop
    y = yon;
elseif t >= T_low_start && t < T_low_stop
    y = yoff;
end

== matlab function libc_hmi/Chirpgenerator/steps ==
  data: rsin output; time input; dtsin output; amp input; w0 input; wE input; t0 input; tE input
function [rsin,dtsin] = dt_chirp(time, amp, w0, wE, t0, tE)
%#codegen

%t = mod(time,Tmax);

dtsin = 0; 
rsin  = 0;

if time < t0
    dtsin = amp*w0*cos(w0*time);
    rsin  = amp*sin(w0*time);
elseif time >= t0 && time < tE
    dtsin = amp*cos(time*(w0+(wE-w0)*(time-t0)/(tE-t0)))*( (w0*tE-wE*t0)/(tE-t0)+2*(wE-w0)/(tE-t0)*time);
    rsin  = amp*sin(time*(w0+(wE-w0*(time-t0)/(tE-t0)))); % + (wE-w0*(time-t0)/(tE-t0))*2*pi);
elseif time >=tE
    dtsin = amp*wE*cos(wE*time);
    rsin  = amp*sin(wE*time);
end

== matlab function libc_hmi/DiscreteChirpgenerator/Subsystem/T_total ==
  data: df_ output; Ttot output; df input; fmax input; t0 input; f0 input
function [df_, Ttot] = dt_chirp(df, fmax, t0, f0)
%#codegen

Ttot = ceil(t0*f0)/f0;
df_ = 0;

%debugh = [0];

if fmax > f0
    df_ = abs(df);
    if df_ == 0
        df_ = 0.01;
    end
    fnew = f0*exp(df_/f0);
    while( fnew < fmax)
       Ttot = Ttot + 1/fnew;
       fnew = fnew*exp(df_/fnew);
    end
elseif fmax < f0
    df_ = - abs(df);
    if df_ == 0
        df_ = -0.01;
    end
    fnew = f0*exp(df_/f0);
    while( fnew > fmax)
       Ttot = Ttot + 1/fnew;
       fnew = fnew*exp(df_/fnew);
    end
end    

Ttot = Ttot + 1/(fmax);

== matlab function libc_hmi/DiscreteChirpgenerator/steps ==
  data: y output; time input; df input; fmax input; t0 input; f input; dy output; t0_next output; f_next output
function [y,dy,t0_next,f_next] = dt_chirp(time, df, fmax, t0, f)%(time, amp, w0, wE, t0, tE)
%#codegen

t0_next = t0;
f_next = f;

if time >= t0_next + 1/f_next % period completed, new frequency
    t0_next = t0_next + 1/f_next;
    if df > 0 % increasing frequency
        %fnew = f*exp(df);
        fnew = f*exp(df/f); % frequenz-abhängige Skalierung
        if fnew <= fmax
            f_next = fnew;
        elseif f < fmax
            f_next = fmax;
        end
    else % decreasing frequency
        %fnew = f*exp(df);
        fnew = f*exp(df/f); % frequenz-abhängige Skalierung
        if fnew >= fmax
            f_next = fnew;
        elseif f > fmax
            f_next = fmax;
        end
    end
end


y  = sin((time-t0_next)*f_next*2*pi);
dy = cos((time-t0_next)*f_next*2*pi)*f_next*2*pi;

== matlab function libc_hmi/DiscreteLinearChirpgenerator/T_total ==
  data: dfc output; Ttot output; df input; fmax input; t0 input; f0 input
function [dfc, Ttot] = dt_chirp(df, fmax, t0, f0)
%#codegen

T1 =ceil(t0*f0);
Ttot = T1;
i=0;
dfc = 0;
if fmax > f0
    while(i*df+f0<fmax)
       Ttot = Ttot + 1/(i*df+f0);
       i=i+1; 
    end
    dfc = abs(df);
elseif fmax < f0
    while(-i*abs(df)+f0 > fmax)
       Ttot = Ttot - 1/(-i*abs(df)+f0);
       i=i+1; 
    end
    dfc = -abs(df);
end
Ttot = Ttot + 1/(fmax);

== matlab function libc_hmi/DiscreteLinearChirpgenerator/steps ==
  data: y output; time input; df input; fmax input; t0 input; f input; dy output; t0_next output; f_next output
function [y,dy,t0_next,f_next] = dt_chirp(time, df, fmax, t0, f)%(time, amp, w0, wE, t0, tE)
%#codegen

%t = mod(time,Tmax);

t0_next = t0;
f_next = f;
if time >= t0_next + 1/f_next
    t0_next = t0_next + 1/f_next;
    if df > 0
        if f+df <= fmax
            f_next = f + df;
        elseif f < fmax
            f_next = fmax;
        end
    else
        if f+df >= fmax
            f_next = f + df;
        elseif f > fmax
            f_next = fmax;
        end
    end
else
    
end

y  = sin((time-t0_next)*f_next*2*pi);
dy = cos((time-t0_next)*f_next*2*pi)*f_next*2*pi;

== matlab function libc_hmi/NewChirpgenerator/ChirpWithWindowTransition ==
  data: asin output; time input; dasin output; amp0 input; ampE input; w0 input; wE input; t0 input; tE input; docutoff_amp input; docutoff_freq input; expfac_amp input; expfac_freq input; instFreq output; damp output
function [asin,dasin,instFreq,damp] = dt_chirp(time, amp0, ampE, w0, wE, t0, tE, docutoff_amp, docutoff_freq, expfac_amp, expfac_freq)

%#codegen
expfac_freq = max(0.1,expfac_freq); % muss für die Ableitung echt größer als 0 sein (bei 1 linearer Anstieg. Falls konstant, wähle wE=w0)
expfac_amp  = max(0.1,expfac_amp);  % muss für die Ableitung echt größer als 0 sein (bei 1 linearer Anstieg)

tE = max(tE,t0+0.1); % 0.1s min. Zeitdifferenz

if amp0 == ampE
    amp = amp0;
    damp = 0;
else
    if (time <= t0) % && docutoff_amp  % <= wichtig, bei time=t0 sonst später -Inf
        amp = amp0;
        damp = 0;
    elseif (time > tE) && docutoff_amp
        amp = ampE;
        damp = 0;
    else
        % Linear Amplitude (positive oder negative Steigung)
        % damp = (ampE-amp0)/(tE-t0);
        % amp = damp*(time-t0)+amp0;
        
        % General Exponential Frequency
        % damp = -Inf at time=t0 (0^(-x))  -->  daher oben time <= t0 statt time < t0
        amp  = (ampE-amp0) *                        ((time-t0)/(tE-t0))^(expfac_amp)  + amp0;
        damp = (ampE-amp0) * expfac_amp * 1/(tE-t0)*((time-t0)/(tE-t0))^(expfac_amp-1);  
        %if expfac_amp <= 1 % Unstetiger Übergang bei t=t0. Extrem bei expfac_amp < 1, aber auch noch etwas bei expfac_amp >= 1
            dT=(tE-t0)/100/expfac_amp; % Bereich des weichen Übergangs. Je breiter desto kleiner expfac_amp.
            if time-t0 <= dT
                damp = damp*(time-t0)/dT; % Interpolation zwischen 0 und damp
            end            
        %end
    end
end

if w0 == wE
    instFreq = w0;
    fsin = sin(instFreq*time);
    dfsin = cos(instFreq*time)*instFreq;
else
    if (time < t0) % && docutoff_freq
        instFreq = w0;
        fsin = sin(instFreq*time);
        dfsin = cos(instFreq*time)*instFreq;
    elseif (time > tE) && docutoff_freq
        fsin = sin(wE*(time-tE) + 1/(expfac_freq+1)*(wE-w0)*(tE-t0) + w0*tE);
        dfsin = cos(wE*(time-tE) + 1/(expfac_freq+1)*(wE-w0)*(tE-t0) + w0*tE)*wE;
        instFreq = wE;
    else
        % Linear Frequency (positive oder negative Steigung)
        % freqSlope = (wE-w0)/(tE-t0);
        % instFreq = freqSlope*(time-t0) + w0;
        % instPhase = 0.5*freqSlope*(time-t0)^2 + w0*time;
        
        % General Exponential Frequency
        dt = tE-t0;
        instFreq  = (wE-w0)*((time-t0)/dt).^expfac_freq + w0;
        instPhase = 1/(expfac_freq+1)*(wE-w0)*((time-t0)/dt).^expfac_freq*(time-t0) + w0*time;
        
        fsin = sin(instPhase);
        dfsin = cos(instPhase)*instFreq;
    end
end

asin = amp*fsin;
dasin = amp*dfsin + damp*fsin;

== matlab function libc_hmi/XYZ-Generator/Dreieck ==
  data: t input; t2 input; x0 input; z0 input; x output; x1 input; t1 input; z2 input; z output
function [x, z] = dreieck(t,t2,x0,z0,x1,t1,z2)

t = rem(t,t2);
if t<t1
    x = (x1-x0)*t/t1+x0;
    z = z0;
else
	x = (x1-x0)*(t2-t)/(t2-t1)+x0;
    z = (z2-z0)*(1-abs(2*(t2-t)/(t2-t1)-1))+z0;
end

% figure(1);clf;
% t = linspace(0,t1);
% plot((x1-x0)*t/t1+x0,z0+t*0);
% hold on;
% t = linspace(t1,t2);
% plot((x1-x0)*(t2-t)/(t2-t1)+x0,(z2-z0)*(1-abs(2*(t2-t)/(t2-t1)-1))+z0);



%#codegen
